simulink model "InvertedPendulum_simonly"  (R2025a)
settings: Solver=ode1  StartTime=0.0  StopTime=80  FixedStep=0.002  RelTol=1e-3  EnableMultiTasking=on
undefined symbols (not defined in the file): A1, B1, C1, D1
libraries: simulink_extras x4
settings Model: SimulationMode=external  ExtModeTrigDuration=50000  Creator=MLevis  LastModifiedBy=User
settings SolverCC: AlgebraicLoopSolver=TrustRegion  PositivePriorityOrder=on
settings DataIOCC: LimitDataPoints=on  SaveFormat=Array  SignalLoggingSaveFormat=ModelDataLogs  ReturnWorkspaceOutputs=off
settings OptimizationCC: ExpressionDepthLimit=2147483647.0  LifeSpan=inf
settings DebuggingCC: UnderspecifiedInitializationDetection=Classic  MergeDetectMultiDrivingBlocksExec=none  SolverPrmCheckMsg=warning  FcnCallInpInsideContextMsg=warning  UnconnectedInputMsg=warning  UnconnectedOutputMsg=warning  UnconnectedLineMsg=warning  StateNameClashWarn=warning  SFUnexpectedBacktrackingDiag=warning  SFNoUnconditionalDefaultTransitionDiag=warning  SFExecutionAtInitializationDiag=none  ArithmeticOperatorsInVariantConditions=warning
settings HardwareCC: ProdBitPerPointer=32.0  ProdBitPerSizeT=32.0  ProdBitPerPtrDiffT=32.0  ProdLargestAtomicFloat=None  ProdIntDivRoundTo=Undefined  ProdEndianess=Unspecified  ProdWordSize=32.0  ProdHWDeviceType=32-bit Generic
settings ModelReferenceCC: EnableRefExpFcnMdlSchedulingChecks=on  PropagateSignalLabelsOutOfModel=off
settings SFSimCC: SimUseLocalCustomCode=off  CustomCodeUndefinedFunction=UseInterfaceOnly
settings RTWCC: SystemTargetFile=quarc_win64.tlc  TemplateMakefile=quarc_default_tmf  RTWUseLocalCustomCode=off  GPUComputeCapability=3.5  Description=QUARC Win64 Target
settings CodeAppCC: StateflowObjectComments=on
settings STFCustomTargetCC: SystemTargetFile=quarc_win64.tlc  TargetPreCompLibLocation=C:\PROGRA~3\QUARC\lib\2017a\win64\release  MultiwordLength=2048.0  DynamicStringBufferSize=256.0  ConcurrentExecutionCompliant=on  DownloadToTarget=on  StopOnOverrun=off  Debug=off
settings GRTTargetCC: ExtMode=on  ExtModeMexFile=quarc_comm  TargetPreCompLibLocation=C:\PROGRA~3\QUARC\lib\2017a\win64\release  TargetLangStandard=C89/C90 (ANSI)  ParMdlRefBuildCompliant=off  CompOptLevelCompliant=off  CombineOutputUpdateFcns=off  MatFileLogging=off  CPPClassGenCompliant=off  GRTInterface=on  UseToolchainInfoCompliant=off
settings ConfigComp: CovMetricSettings=dw  CovSaveCumulativeToWorkspaceVar=on  CovSaveSingleToWorkspaceVar=on  CovExternalEMLEnable=off  CovSFcnEnable=off

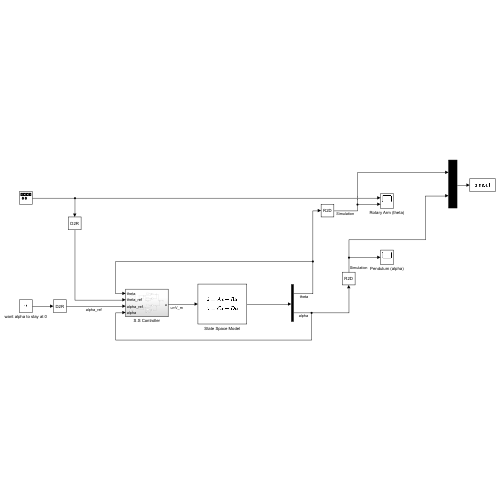
[thumbnail: Simulink's stored preview of the top-level diagram]
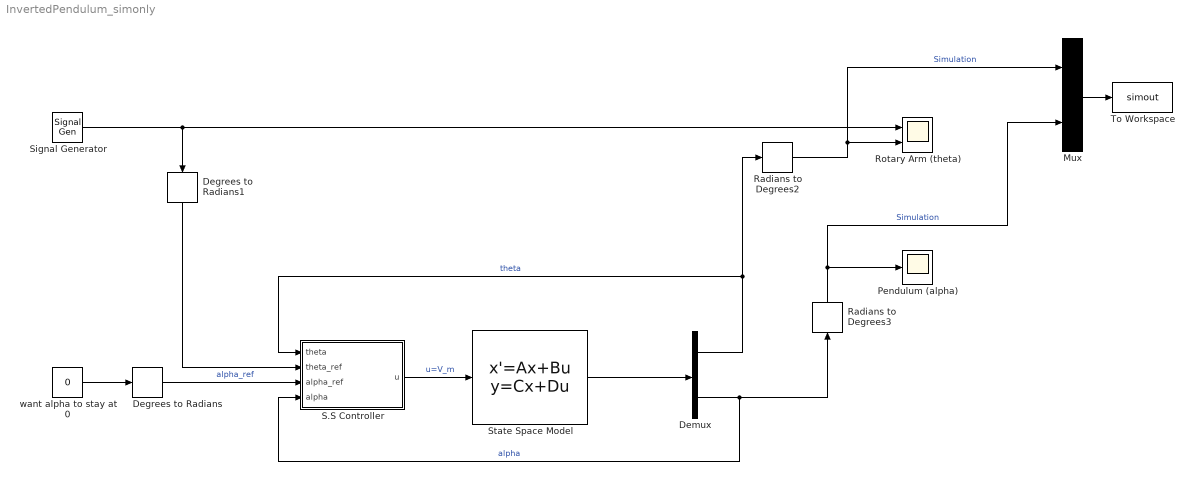
== system InvertedPendulum_simonly ==
  Degrees to Radians : simulink_extras/Transformations/Degrees to Radians
  Degrees to Radians1 : simulink_extras/Transformations/Degrees to Radians
  Demux : Demux  Outputs=2
  Mux : Mux  Inputs=2
  Pendulum (alpha) : Scope
      settings: TimeSpan=40  ActiveDisplayYMinimum=-3.3019305477952603  ActiveDisplayYMaximum=1.7771573134348111  DataLoggingMaxPoints=50000
  Radians to Degrees2 : simulink_extras/Transformations/Radians to Degrees
  Radians to Degrees3 : simulink_extras/Transformations/Radians to Degrees
  Rotary Arm (theta) : Scope  NumInputPorts=2
      settings: TimeSpan=40  ActiveDisplayYMinimum=14.205263557699302  ActiveDisplayYMaximum=32.787111339958081  DataLoggingMaxPoints=50000
  S.S Controller : Subsystem
  Signal Generator : SignalGenerator  WaveForm=square  Amplitude=25  Frequency=0.05
  State Space Model : StateSpace  A=A1  B=B1  C=C1  D=D1  InitialCondition=0
  To Workspace : ToWorkspace  VariableName=simout  SaveFormat=Structure With Time  SampleTime=-1
  want alpha to stay at 0 : Constant  Value=0
  wires:
  Signal Generator/1 -> Degrees to Radians1/1, Rotary Arm (theta)/1
  Mux/1 -> To Workspace/1
  Demux/2 -> S.S Controller/4(alpha), Radians to Degrees3/1  "alpha"
  State Space Model/1 -> Demux/1
  Demux/1 -> S.S Controller/1(theta), Radians to Degrees2/1  "theta"
  Radians to Degrees2/1 -> Mux/1, Rotary Arm (theta)/2  "Simulation"
  Radians to Degrees3/1 -> Mux/2, Pendulum (alpha)/1  "Simulation"
  S.S Controller/1(u) -> State Space Model/1  "u=V_m"
  Degrees to Radians1/1 -> S.S Controller/2(theta_ref)
  want alpha to stay at 0/1 -> Degrees to Radians/1
  Degrees to Radians/1 -> S.S Controller/3(alpha_ref)  "alpha_ref"

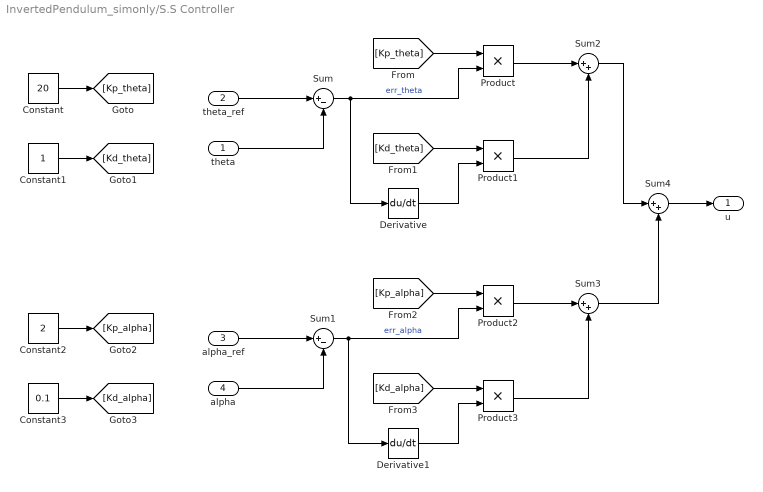
== system InvertedPendulum_simonly/S.S Controller ==
  theta : Inport
  theta_ref : Inport  Port=2
  alpha_ref : Inport  Port=3
  alpha : Inport  Port=4
  Constant : Constant  Value=20
  Constant1 : Constant
  Constant2 : Constant  Value=2
  Constant3 : Constant  Value=0.1
  Derivative : Derivative
  Derivative1 : Derivative
  Product{,1..3} (4 alike) : Product
  Sum : Sum  Inputs=|+-
  Sum1 : Sum  Inputs=|+-
  Sum2 : Sum  Inputs=|++
  Sum3 : Sum  Inputs=|++
  Sum4 : Sum  Inputs=|++
  u : Outport
  wires:
  alpha_ref/1 -> Sum1/1
  alpha/1 -> Sum1/2
  Constant/1 -> [Kp_theta]
  Constant1/1 -> [Kd_theta]
  [Kp_theta] -> Product/1
  Sum/1 -> Product/2, Derivative/1  "err_theta"
  [Kd_theta] -> Product1/1
  Derivative/1 -> Product1/2
  Constant2/1 -> [Kp_alpha]
  Constant3/1 -> [Kd_alpha]
  [Kd_alpha] -> Product3/1
  [Kp_alpha] -> Product2/1
  Derivative1/1 -> Product3/2
  Sum1/1 -> Product2/2, Derivative1/1  "err_alpha"
  Product/1 -> Sum2/1
  Product1/1 -> Sum2/2
  Product2/1 -> Sum3/1
  Product3/1 -> Sum3/2
  Sum4/1 -> u/1
  Sum3/1 -> Sum4/2
  Sum2/1 -> Sum4/1
  theta_ref/1 -> Sum/1
  theta/1 -> Sum/2
